simulink model "average_example"  (Simulink 7.6)
settings: Solver=ode45  StartTime=0.0  StopTime=24*3600  MaxStep=60  RelTol=1e-3
libraries: carnot x1
settings Model: Creator=drhf  LastModifiedBy=drhf

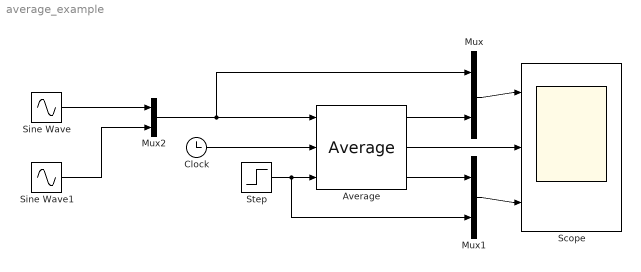
== system average_example ==
  Average : carnot/Toolbox/Average  SystemSampleTime=-1  time_intervall=1 h  offset_flag=on  enable_flag=on
  Clock : Clock
      settings: Decimation=10
  Mux : Mux  Inputs=2
  Mux1 : Mux  Inputs=2
  Mux2 : Mux  Inputs=2
  Scope : Scope  NumInputPorts=3
      settings: YMin=-5~-5~-5  YMax=5~5~5
  Sine Wave : Sin  Frequency=2*pi/(24*3600)  SampleTime=0
  Sine Wave1 : Sin  Frequency=2*pi/(24*3600)  Phase=3*3600  SampleTime=0
  Step : Step  Time=3600  SampleTime=0
  wires:
  Sine Wave/1 -> Mux2/1
  Clock/1 -> Average/2
  Step/1 -> Average/3, Mux1/2
  Average/2 -> Scope/2
  Average/1 -> Mux/2
  Mux/1 -> Scope/1
  Average/3 -> Mux1/1
  Mux1/1 -> Scope/3
  Mux2/1 -> Average/1, Mux/1
  Sine Wave1/1 -> Mux2/2
